simulink model "stage"  (R2020a)
settings: Solver=FixedStepDiscrete  StartTime=0.0  StopTime=10.0  RelTol=1e-3
settings Model: Creator=thomas  LastModifiedBy=thomas

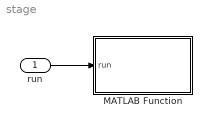
== system stage ==
  run : Inport  OutDataTypeStr=boolean
  MATLAB Function : MATLAB Function  TreatAsAtomicUnit=on
  wires:
  run/1 -> MATLAB Function/1(run)

== matlab function stage/MATLAB Function ==
  data: run input
function stage(run)
    coder.extrinsic('evalin');
    if run
        evalin('base', 'vessel_control.activateNextStage();');
    end
end
